simulink subsystem "mean2"  (R2022a)
settings: Solver=VariableStepAuto  StartTime=0.0  StopTime=10.0  RelTol=1e-3
undefined symbols (not defined in the file or in its folder): NumBits1, NumBits2, Slope1, Slope2
libraries: simulink x1
settings Model: Creator=dileepan  LastModifiedBy=dileepan
settings DebuggingCC: UnconnectedInputMsg=warning  UnconnectedOutputMsg=warning  UnconnectedLineMsg=warning
settings RTWCC: DLArmComputeVersion=19.05

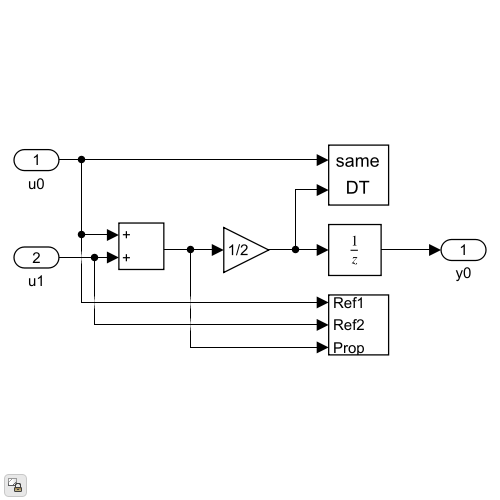
[thumbnail: Simulink's stored preview of the top-level diagram]
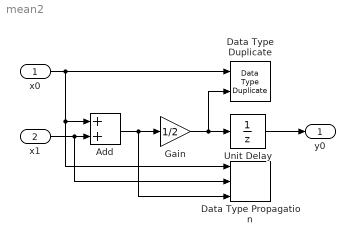
== system mean2 ==
  x0 : Inport
  x1 : Inport  Port=2
  Add : Sum  OutDataTypeStr=Inherit: Inherit via back propagation
  Data Type Duplicate : DataTypeDuplicate
  Data Type Propagation : simulink/Signal Attributes/Data Type Propagation  PropDataType=fixdt(1, 16)  IfRefDouble=double  IfRefSingle=single  IsSigned=IsSigned1 or IsSigned2  NumBitsBase=max([NumBits1 NumBits2])  NumBitsMult=1  NumBitsAdd=1  NumBitsAllowFinal=1:64  PropScaling=2^-10  ValuesUsedBestPrec=[5 -7]  SlopeBase=min([Slope1 Slope2])  SlopeMult=1  SlopeAdd=0  BiasBase=Bias1  BiasMult=1  BiasAdd=0
      settings: SourceProductBaseCode=SL
  Gain : Gain  Gain=1/2  OutDataTypeStr=Inherit: Inherit via back propagation  RndMeth=Round
  Unit Delay : UnitDelay  SampleTime=-1  HasFrameUpgradeWarning=on
  y0 : Outport
  wires:
  Add/1 -> Data Type Propagation/3, Gain/1
  Unit Delay/1 -> y0/1
  x1/1 -> Data Type Propagation/2, Add/2
  x0/1 -> Data Type Duplicate/1, Data Type Propagation/1, Add/1
  Gain/1 -> Data Type Duplicate/2, Unit Delay/1
